simulink model "master_task"  (Simulink 7.1)
libraries: mathlib x9, inoutlib x3
settings Model: Creator=jsobota  LastModifiedBy=jsobota  ExtModeTrigMode=oneshot  ExtModeArmWhenConnect=off

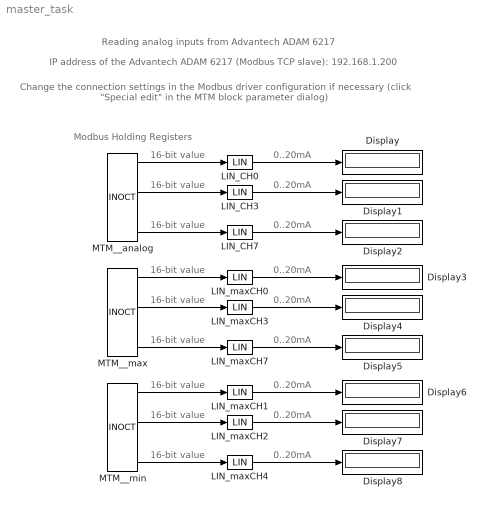
== system master_task ==
  note: Change the connection settings in the Modbus driver configuration
      | if necessary (click "Special edit" in the MTM block parameter dialog)
  note: Modbus Holding Registers
  note: IP address of the Advantech ADAM 6217 (Modbus TCP slave): 192.168.1.200
  note: 16-bit value
  note: 0..20mA
  note: 16-bit value
  note: 0..20mA
  note: 16-bit value
  note: 0..20mA
  note: 16-bit value
  note: 0..20mA
  note: 16-bit value
  note: 0..20mA
  note: 16-bit value
  note: 0..20mA
  note: 16-bit value
  note: 0..20mA
  note: 16-bit value
  note: 0..20mA
  note: 16-bit value
  note: 0..20mA
  note: Reading analog inputs from Advantech ADAM 6217
  Display{,1..8} (9 alike) : Display
      settings: Format=Best fit
  LIN_CH0 : mathlib/LIN  u1=0  y1=0  u2=65535  y2=20
  LIN_CH3 : mathlib/LIN  u1=0  y1=0  u2=65535  y2=20
  LIN_CH7 : mathlib/LIN  u1=0  y1=0  u2=65535  y2=20
  LIN_maxCH{0..4,7} (6 alike) : mathlib/LIN  u1=0  y1=0  u2=65535  y2=20
  MTM__analog : inoutlib/INOCT
  MTM__max : inoutlib/INOCT
  MTM__min : inoutlib/INOCT
  wires:
  LIN_CH0/1 -> Display/1
  LIN_CH3/1 -> Display1/1
  LIN_CH7/1 -> Display2/1
  LIN_maxCH0/1 -> Display3/1
  LIN_maxCH1/1 -> Display6/1
  LIN_maxCH2/1 -> Display7/1
  LIN_maxCH3/1 -> Display4/1
  LIN_maxCH4/1 -> Display8/1
  LIN_maxCH7/1 -> Display5/1
  MTM__analog/1 -> LIN_CH0/1
  MTM__analog/4 -> LIN_CH3/1
  MTM__analog/8 -> LIN_CH7/1
  MTM__max/1 -> LIN_maxCH0/1
  MTM__max/4 -> LIN_maxCH3/1
  MTM__max/8 -> LIN_maxCH7/1
  MTM__min/1 -> LIN_maxCH1/1
  MTM__min/4 -> LIN_maxCH2/1
  MTM__min/8 -> LIN_maxCH4/1
